simulink model "spring_damperSIM"  (R2015a)
settings: Solver=ode45  StartTime=0.0  StopTime=10.0  RelTol=1e-3
values from neighbouring files (symbols this model uses):
  b = 0.1    [motor.m]    (also in spring_damper.m = 2)
  k = 0.01    [motor.m]    (also in spring_damper.m = 1)
  m = 1    [spring_damper.m]
settings Model: Creator=ahmed alaa  LastModifiedBy=ahmed alaa

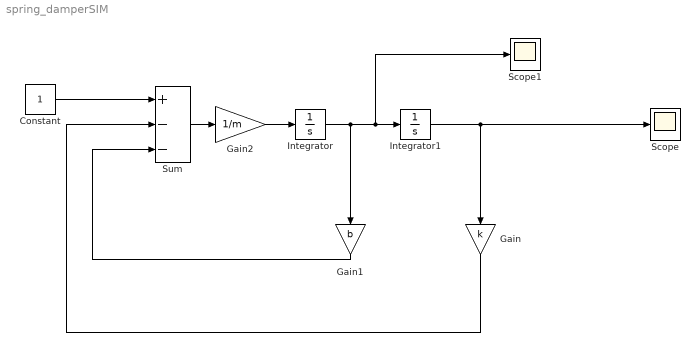
== system spring_damperSIM ==
  Constant : Constant
  Gain : Gain  Gain=k
  Gain1 : Gain  Gain=b
  Gain2 : Gain  Gain=1/m
  Integrator : Integrator
  Integrator1 : Integrator
  Scope : Scope
  Scope1 : Scope
  Sum : Sum  Inputs=+--
  wires:
  Sum/1 -> Gain2/1
  Integrator/1 -> Scope1/1, Integrator1/1, Gain1/1
  Integrator1/1 -> Scope/1, Gain/1
  Gain/1 -> Sum/2
  Gain1/1 -> Sum/3
  Constant/1 -> Sum/1
  Gain2/1 -> Integrator/1
